simulink model "Tarea_4_1"  (R2021a)
settings: Solver=VariableStepAuto  StartTime=0.0  StopTime=100.0  RelTol=1e-3
values from neighbouring files (symbols this model uses):
  sigma = 0.01    [Tarea_4_v2.m]
libraries: dspsrcs4 x1
settings Model: Creator=Seb  LastModifiedBy=Seb

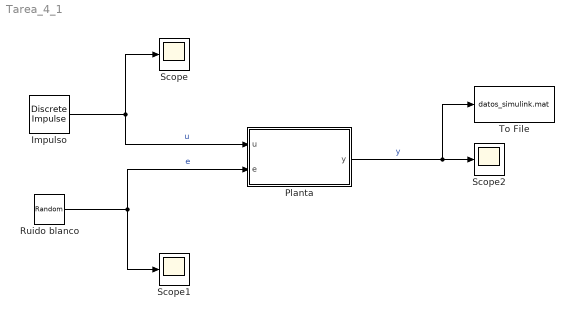
== system Tarea_4_1 ==
  Impulso : dspsrcs4/Discrete  Impulse  Delay=0  SampleTime=1  FrameSample=1  OutputFrames=off  dataType=double  isSigned=on  wordLen=16  udDataType=sfix(16)  fracBitsMode=Best precision  numFracBits=15  OutDataTypeStr=double  LastOutDataTypeStr=double
  Planta : Subsystem
  Ruido blanco : RandomNumber  Variance=sigma^2  Seed=7  SampleTime=1
  Scope : Scope
  Scope1 : Scope
  Scope2 : Scope
  To File : ToFile  Filename=datos_simulink.mat  MatrixName=y  SampleTime=1
  wires:
  Ruido blanco/1 -> Planta/2(e), Scope1/1  "e"
  Impulso/1 -> Planta/1(u), Scope/1  "u"
  Planta/1(y) -> To File/1, Scope2/1  "y"

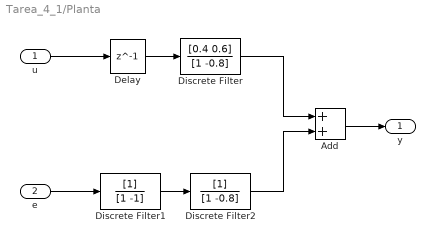
== system Tarea_4_1/Planta ==
  u : Inport
  e : Inport  Port=2
  Add : Sum
  Delay : Delay  DelayLength=1  InitialCondition=0
  Discrete Filter : DiscreteFilter  Numerator=[0.4 0.6]  Denominator=[1 -0.8]  SampleTime=1
  Discrete Filter1 : DiscreteFilter  Denominator=[1 -1]  SampleTime=1
  Discrete Filter2 : DiscreteFilter  Denominator=[1 -0.8]  SampleTime=1
  y : Outport
  wires:
  Add/1 -> y/1
  u/1 -> Delay/1
  Discrete Filter1/1 -> Discrete Filter2/1
  e/1 -> Discrete Filter1/1
  Discrete Filter/1 -> Add/1
  Discrete Filter2/1 -> Add/2
  Delay/1 -> Discrete Filter/1
